simulink model "non_linear_tank"  (R2020a)
settings: Solver=VariableStepAuto  StartTime=0.0  StopTime=sim_time  RelTol=1e-3
undefined symbols (not defined in the file): k1, k2, p, r, x1_0, x2_0
settings Model: Creator=jakelangton  LastModifiedBy=jakelangton

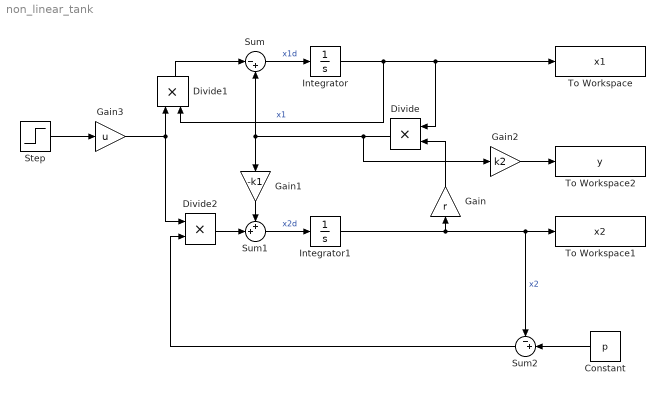
== system non_linear_tank ==
  Constant : Constant  Value=p
  Divide : Product  Inputs=**
  Divide1 : Product  Inputs=**
  Divide2 : Product  Inputs=**
  Gain : Gain  Gain=r
  Gain1 : Gain  Gain=-k1
  Gain2 : Gain  Gain=k2
  Gain3 : Gain  Gain=u
  Integrator : Integrator  InitialCondition=x1_0
  Integrator1 : Integrator  InitialCondition=x2_0
  Step : Step  Before=1  SampleTime=0
  Sum : Sum  Inputs=|-+
  Sum1 : Sum  Inputs=++|
  Sum2 : Sum  Inputs=-+|
  To Workspace : ToWorkspace  VariableName=x1  SaveFormat=Timeseries  SampleTime=-1
  To Workspace1 : ToWorkspace  VariableName=x2  SaveFormat=Timeseries  SampleTime=-1
  To Workspace2 : ToWorkspace  VariableName=y  SaveFormat=Timeseries  SampleTime=-1
  wires:
  Integrator1/1 -> Sum2/1, To Workspace1/1, Gain/1  "x2"
  Gain/1 -> Divide/2
  Integrator/1 -> Divide1/2, To Workspace/1, Divide/1  "x1"
  Sum/1 -> Integrator/1  "x1d"
  Divide/1 -> Gain2/1, Sum/2, Gain1/1
  Sum1/1 -> Integrator1/1  "x2d"
  Gain1/1 -> Sum1/1
  Divide1/1 -> Sum/1
  Gain2/1 -> To Workspace2/1
  Step/1 -> Gain3/1
  Constant/1 -> Sum2/2
  Sum2/1 -> Divide2/2
  Divide2/1 -> Sum1/2
  Gain3/1 -> Divide1/1, Divide2/1
